simulink model "practica1validacion"  (R2019b)
settings: Solver=VariableStepAuto  StartTime=0.0  StopTime=10.0  RelTol=1e-3
settings Model: Creator=Usuario  LastModifiedBy=Usuario

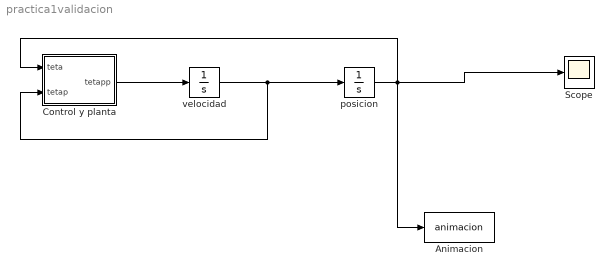
== system practica1validacion ==
  "Animacion " : MATLABFcn  MATLABFcn=animacion  OutputDimensions=0
  Control y planta : MATLAB Function  TreatAsAtomicUnit=on
  Scope : Scope
  posicion : Integrator  InitialCondition=pi/2
  velocidad : Integrator
  wires:
  Control y planta/1(tetapp) -> velocidad/1
  velocidad/1 -> Control y planta/2(tetap), posicion/1
  posicion/1 -> Control y planta/1(teta), Scope/1, "Animacion "/1

== matlab function practica1validacion/Control y planta ==
  data: teta input; tetapp output; tetap input
function tetapp = fcn(teta,tetap)
%%parametros
m = 0.067403827487648046;
lc = 150/1e3+1.3213515470703689/1e3-10/1000;
I = 502.1506615468216/1e6;
g = 9.81;
B=0.0015;
kp = 450;
kd = 10;
tetad=pi/2;
%control
%%e=tetad-teta;
%%tau = kp*e-kd*tetap;
tau=0.05;
%planta
tetapp = 1/(m*lc^2+I)*(tau-m*g*lc*sin(teta)-B*tetap);
